simulink model "kalman_subsystem"  (R2024b)
settings: Solver=VariableStepAuto  StartTime=0.0  StopTime=10.0  RelTol=1e-3
settings Model: Creator=ARULPAVALAN S A  LastModifiedBy=ARULPAVALAN S A

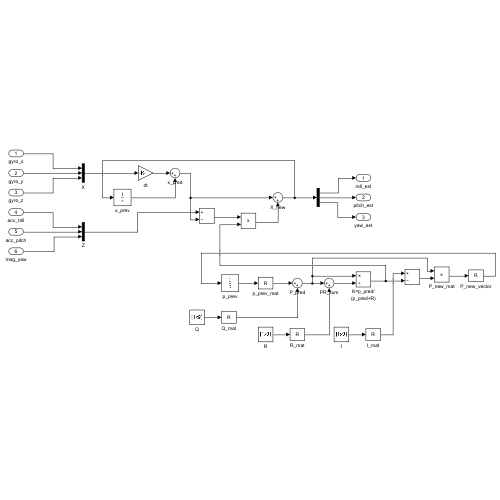
[thumbnail: Simulink's stored preview of the top-level diagram]
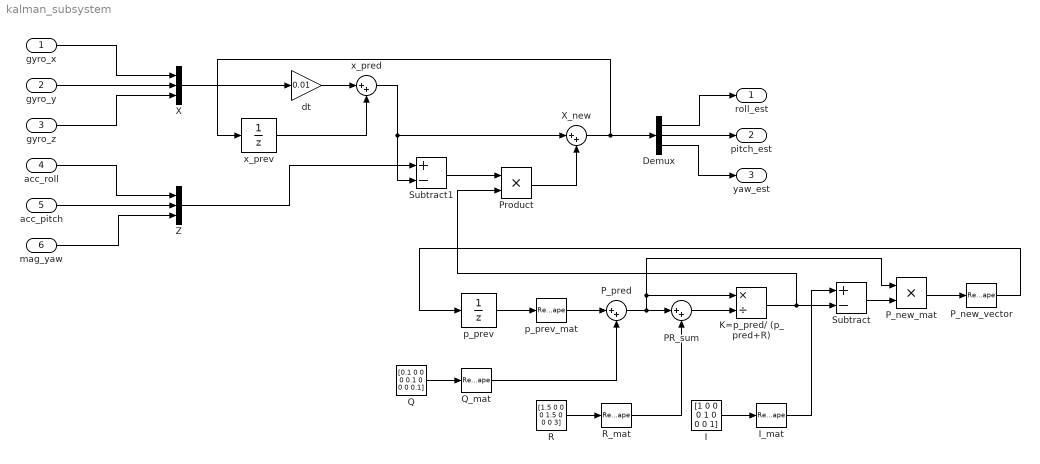
== system kalman_subsystem ==
  gyro_x : Inport
  gyro_y : Inport  Port=2
  gyro_z : Inport  Port=3
  acc_roll : Inport  Port=4
  acc_pitch : Inport  Port=5
  mag_yaw : Inport  Port=6
  Demux : Demux  Outputs=3
  I : Constant  Value=[1 0 0 0 1 0 0 0 1]
  I_mat : Reshape  OutputDimensionality=Customize  OutputDimensions=[3,3]
  K=p_pred/ (p_pred+R) : Product  Inputs=*/
  "PR_sum " : Sum  Inputs=|++
  P_new_mat : Product
  P_new_vector : Reshape  OutputDimensionality=Customize  OutputDimensions=[1,9]
  "P_pred " : Sum  Inputs=|++
  Product : Product
  Q : Constant  Value=[0.1 0 0 0 0.1 0 0 0 0.1]
  Q_mat : Reshape  OutputDimensionality=Customize  OutputDimensions=[3,3]
  R : Constant  Value=[1.5 0 0 0 1.5 0 0 0 3]
  R_mat : Reshape  OutputDimensionality=Customize  OutputDimensions=[3,3]
  Subtract : Sum  Inputs=+-
  Subtract1 : Sum  Inputs=+-
  X : Mux  Inputs=3
  X_new : Sum  Inputs=|++
  Z : Mux  Inputs=3
  dt : Gain  Gain=0.01
  p_prev : UnitDelay  InitialCondition=[1 0 0 0 1 0 0 0 1]  SampleTime=-1  HasFrameUpgradeWarning=on
  p_prev_mat : Reshape  OutputDimensionality=Customize  OutputDimensions=[3,3]
  "x_pred " : Sum  Inputs=|++
  x_prev : UnitDelay  SampleTime=-1  HasFrameUpgradeWarning=on
  roll_est : Outport
  pitch_est : Outport  Port=2
  yaw_est : Outport  Port=3
  wires:
  Demux/2 -> pitch_est/1
  acc_pitch/1 -> Z/2
  gyro_z/1 -> X/3
  gyro_y/1 -> X/2
  R/1 -> R_mat/1
  "x_pred "/1 -> X_new/1, Subtract1/2
  Product/1 -> X_new/2
  gyro_x/1 -> X/1
  dt/1 -> "x_pred "/1
  x_prev/1 -> "x_pred "/2
  P_new_vector/1 -> p_prev/1
  Demux/1 -> roll_est/1
  I/1 -> I_mat/1
  Q/1 -> Q_mat/1
  Demux/3 -> yaw_est/1
  Q_mat/1 -> "P_pred "/2
  I_mat/1 -> Subtract/1
  p_prev_mat/1 -> "P_pred "/1
  X_new/1 -> Demux/1, x_prev/1
  X/1 -> dt/1
  p_prev/1 -> p_prev_mat/1
  K=p_pred/ (p_pred+R)/1 -> Product/2, Subtract/2
  Subtract/1 -> P_new_mat/2
  "PR_sum "/1 -> K=p_pred/ (p_pred+R)/2
  R_mat/1 -> "PR_sum "/2
  "P_pred "/1 -> P_new_mat/1, K=p_pred/ (p_pred+R)/1, "PR_sum "/1
  mag_yaw/1 -> Z/3
  P_new_mat/1 -> P_new_vector/1
  acc_roll/1 -> Z/1
  Z/1 -> Subtract1/1
  Subtract1/1 -> Product/1
